simulink model "Aileron"  (R2023a)
settings: Solver=VariableStepAuto  StartTime=0.0  StopTime=1.5  RelTol=1e-3
model workspace (MAT data in the model file):
  a1 = 0.5
  a2 = 2
  a3 = 2.5
libraries: simulink x1
settings Model: Creator=MY PC  LastModifiedBy=MY PC

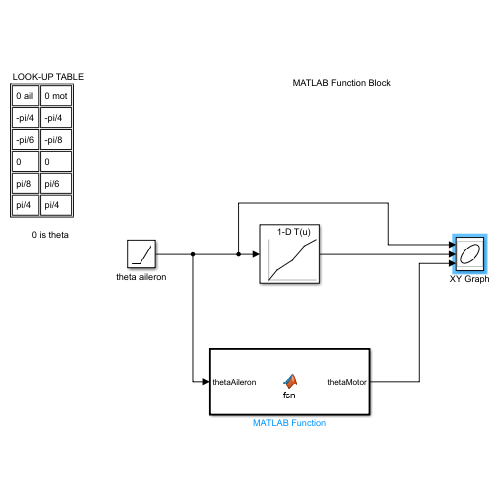
[thumbnail: Simulink's stored preview of the top-level diagram]
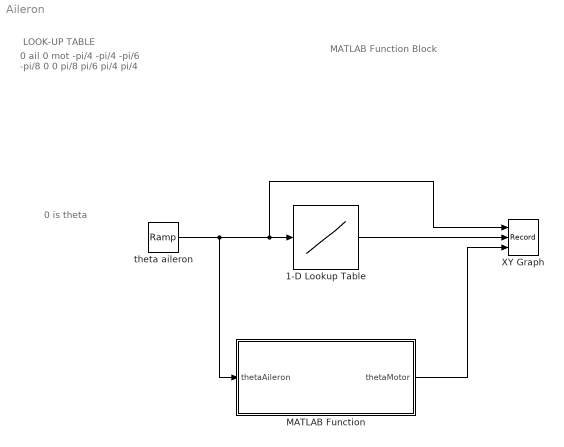
== system Aileron ==
  note: MATLAB Function Block
  note: 0 is theta
  note: LOOK-UP TABLE
  note: 0 ail
      | 0 mot
      |
      | -pi/4
      | -pi/4
      |
      | -pi/6
      | -pi/8
      |
      | 0
      | 0
      |
      | pi/8
      | pi/6
      |
      | pi/4
      | pi/4
  1-D Lookup Table : Lookup_n-D  NumberOfTableDimensions=1  BreakpointsForDimension1=[-pi/4,-pi/6,0,pi/8,pi/4]  Table=[-pi/4,-pi/8,0,pi/6,pi/4]  InternalRulePriority=Speed  RndMeth=Simplest
  MATLAB Function : MATLAB Function  TreatAsAtomicUnit=on
  XY Graph : Record  FileSettingsInternal="{\"entries\":[{\"content\":{\"excelSettings\":{\"content\":{},\"type\":\"Streamout.ExcelSettings\"}},\"type\":\"Streamout.FileSettingStorage\",\"uuid\":\"95d6381d-c6d1-4091-b476-938793d5ec33\"}],\"packageUris\":[\"http://schema.mathworks.com/mf0/streamout_blocks/R2020a\"],\"version\":\"1.0\"}"  Layout=[1 1]  SignalsInternal="{\"entries\":[{\"content\":{\"signals\":[{\"content\":{\"blockPath\":[\"Aileron/XY Graph\"],\"dimensions\":[1],\"domain\":\"Aileron/XY Graph\",\"lineColor\":\"#a2142f\",\"plots\":[1],\"port\":1,\"sid\":[\"\"],\"signalID\":249,\"signalName\":\"theta aileron\"},\"type\":\"RecordBlkView.Signal\",\"uuid\":\"22f1212a-a864-4911-a401-610d4236e8fa\"},{\"content\":{\"blockPath\":[\"Aileron/XY Graph\"],\"dimensions\":[1],\"domain\":\"Aileron/XY Graph\",\"lineColor\":\"#139fff\",\"plots\":[1],\"port\":2,\"sid\":[\"\"],\"signalID\":253,\"signalName\":\"1-D Lookup\\nTable\"},\"type\":\"RecordBlkView.Signal\",\"uuid\":\"ed241102-1d40-4755-9120-7fa30f6abdc4\"},{\"content\":{\"blockPath\":[\"Aileron/XY Graph\"],\"dimensions\":[1],\"domain\":\"Aileron/XY Graph\",\"lineColor\":\"#fe330a\",\"plots\":[1],\"port\":3,\"sid\":[\"\"],\"signalID\":257,\"signalName\":\"MATLAB Function\"},\"type\":\"RecordBlkView.Signal\",\"uuid\":\"5f852d9c-ab44-42eb-b745-54b1c8742bed\"}]},\"type\":\"RecordBlkView.InputSignals\",\"uuid\":\"32ce3e22-d765-4417-926c-5663caf57750\"}],\"packageUris\":[\"http://schema.mathworks.com/mf0/streamout_blocks/R2020a\"],\"version\":\"1.0\"}"  VisualizationBindings="{\"xyplotplugin\":{\"info\":[{\"series\":[{\"bindingParametersList\":[{\"parameter\":\"X-Axis\",\"signalID\":249,\"signalName\":\"theta aileron\"},{\"parameter\":\"Y-Axis\",\"signalID\":253,\"signalName\":\"1-D Lookup\\nTable\"}],\"seriesID\":22843},{\"bindingParametersList\":[{\"parameter\":\"X-Axis\",\"signalID\":249,\"signalName\":\"theta aileron\"},{\"parameter\":\"Y-Axis\",\"signalID\":257,\"signalName\":\"MATLAB Function\"}],\"seriesID\":375}],\"subplotID\":1}]}}"  CompatibilityTag=XY  st=-1
  theta aileron : simulink/Sources/Ramp  slope=1  start=0  InitialOutput=-pi/4
  wires:
  theta aileron/1 -> MATLAB Function/1(thetaAileron), XY Graph/1, 1-D Lookup Table/1
  MATLAB Function/1(thetaMotor) -> XY Graph/3
  1-D Lookup Table/1 -> XY Graph/2

== matlab function Aileron/MATLAB Function ==
  data: thetaAileron input; thetaMotor output; a3 parameter; a2 parameter; a1 parameter
function thetaMotor = fcn(thetaAileron, a3, a2, a1)

thetaMotor = a1*thetaAileron*(a2*thetaAileron^2 + a3*thetaAileron^4);
